simulink model "Automatic_Cruise_control"  (R2020b)
settings: Solver=VariableStepAuto  StartTime=0.0  StopTime=10  RelTol=1e-3
undefined symbols (not defined in the file): b, J, K, ki, kp, L, m, R
settings Model: Creator=intel  LastModifiedBy=intel
settings DebuggingCC: ModelReferenceExtraNoncontSigs=warning

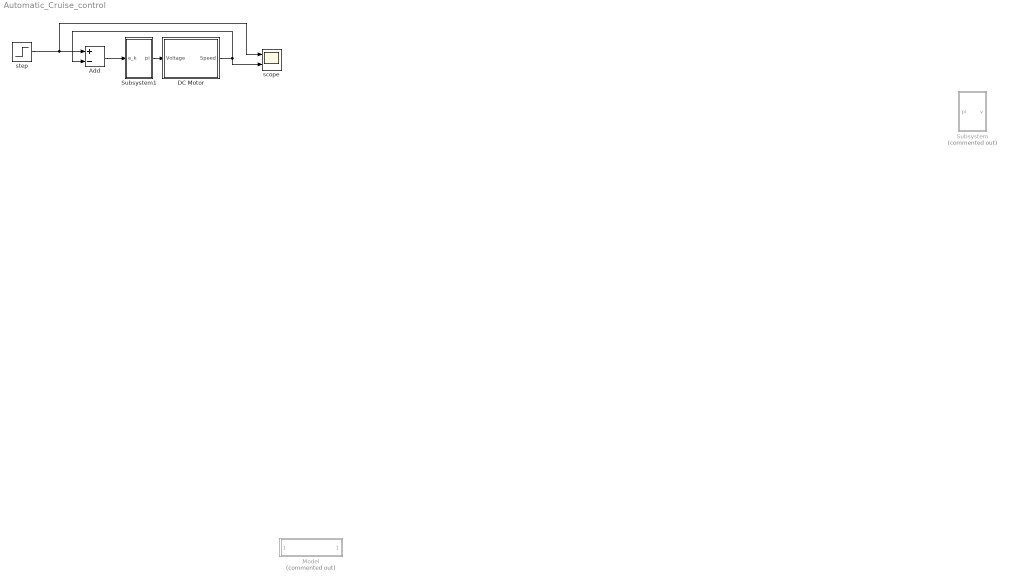
== system Automatic_Cruise_control ==
  Add : Sum  Inputs=+-
  DC Motor : Subsystem
  Model : ModelReference  Commented=on  ModelNameDialog=picntrl.slx  ModelReferenceVersion=1.3
  Subsystem : Subsystem  Commented=on
  Subsystem1 : Subsystem
  scope : Scope  NumInputPorts=2
  step : Step  After=u  SampleTime=0
  wires:
  step/1 -> scope/1, Add/1
  Add/1 -> Subsystem1/1(e_k)
  Subsystem1/1(pi) -> DC Motor/1(Voltage)
  DC Motor/1(Speed) -> scope/2, Add/2

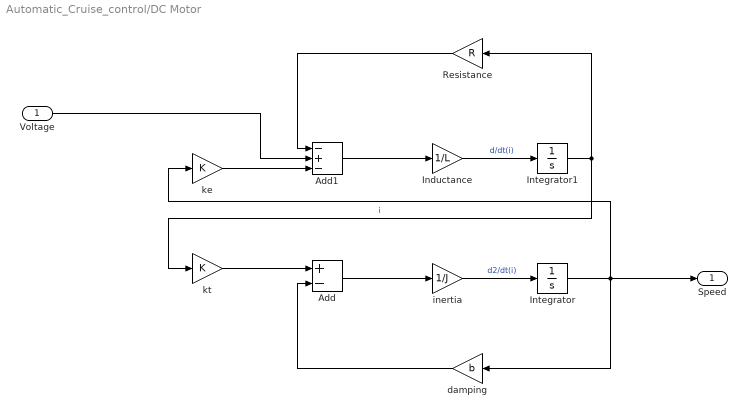
== system Automatic_Cruise_control/DC Motor ==
  Voltage : Inport
  Add : Sum  Inputs=+-
  Add1 : Sum  Inputs=-+-
  Inductance : Gain  Gain=1/L
  Integrator : Integrator
  Integrator1 : Integrator
  Resistance : Gain  Gain=R
  damping : Gain  Gain=b
  inertia : Gain  Gain=1/J
  ke : Gain  Gain=K
  kt : Gain  Gain=K
  Speed : Outport
  wires:
  Integrator/1 -> Speed/1, ke/1, damping/1
  ke/1 -> Add1/3
  Voltage/1 -> Add1/2
  Inductance/1 -> Integrator1/1  "d/dt(i)"
  Integrator1/1 -> Resistance/1, kt/1  "i"
  damping/1 -> Add/2
  Add/1 -> inertia/1
  Resistance/1 -> Add1/1
  Add1/1 -> Inductance/1
  inertia/1 -> Integrator/1  "d2/dt(i)"
  kt/1 -> Add/1

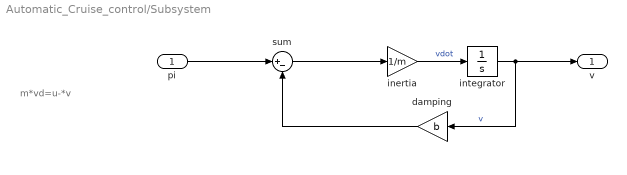
== system Automatic_Cruise_control/Subsystem ==
  note: m*vd=u-*v
  pi : Inport
  damping : Gain  Gain=b
  inertia : Gain  Gain=1/m
  integrator : Integrator
  sum : Sum  Inputs=|+-
  v : Outport
  wires:
  damping/1 -> sum/2
  integrator/1 -> v/1, damping/1  "v"
  sum/1 -> inertia/1
  pi/1 -> sum/1
  inertia/1 -> integrator/1  "vdot"

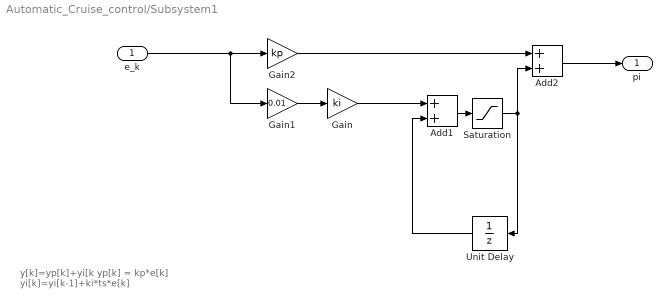
== system Automatic_Cruise_control/Subsystem1 ==
  note: y[k]=yp[k]+yi[k
      | yp[k] = kp*e[k]
      | yi[k]=yi[k-1]+ki*ts*e[k]
  e_k : Inport  OutDataTypeStr=double  PortDimensions=1  SampleTime=0
  Add1 : Sum
  Add2 : Sum
  Gain : Gain  Gain=ki
  Gain1 : Gain  Gain=0.01
  Gain2 : Gain  Gain=kp
  Saturation : Saturate  UpperLimit=1  LowerLimit=-1
  Unit Delay : UnitDelay  SampleTime=-1  HasFrameUpgradeWarning=on
  pi : Outport  OutDataTypeStr=double  PortDimensions=1  SampleTime=0
  wires:
  Saturation/1 -> Unit Delay/1, Add2/2
  e_k/1 -> Gain2/1, Gain1/1
  Unit Delay/1 -> Add1/2
  Add2/1 -> pi/1
  Gain2/1 -> Add2/1
  Gain1/1 -> Gain/1
  Gain/1 -> Add1/1
  Add1/1 -> Saturation/1
